simulink model "UAV_dinamica_pqr"  (R2014b)
settings: Solver=ode45  StartTime=0.0  StopTime=10.0  RelTol=1e-3
values from neighbouring files (symbols this model uses):
  Ir = 1e-3    (= 0.001)    [main_model1.m]    (also in main_model2.m; main_modelo_linear_v1.m = 0.01; main_modelo_linear_v2.m = 0.01; main_modelo_nao_linear_v1.m)
  Ixx = 1e-2    (= 0.01)    [main_model1.m]    (also in main_model2.m; main_modelo_linear_v1.m; main_modelo_linear_v2.m; main_modelo_nao_linear_v1.m)
  Iyy = 1e-2    (= 0.01)    [main_model1.m]    (also in main_model2.m; main_modelo_linear_v1.m; main_modelo_linear_v2.m; main_modelo_nao_linear_v1.m)
  Izz = 1.8e-2    (= 0.018)    [main_model1.m]    (also in main_model2.m; main_modelo_linear_v1.m; main_modelo_linear_v2.m; main_modelo_nao_linear_v1.m)
  Kd_rot = 0.01    [main_model1.m]    (also in main_model2.m; main_modelo_linear_v1.m = 0; main_modelo_linear_v2.m = 0; main_modelo_nao_linear_v1.m)
  Ki_rot = 1.0    (= 1)    [main_model1.m]    (also in main_model2.m; main_modelo_linear_v1.m = 0.5; main_modelo_linear_v2.m = 0.5; main_modelo_nao_linear_v1.m)
  Kp_rot = 10    [main_model1.m]    (also in main_model2.m; main_modelo_linear_v1.m = 1; main_modelo_linear_v2.m = 1; main_modelo_nao_linear_v1.m)
  p0 = 0    [main_model2.m]    (also in main_modelo_linear_v1.m; main_modelo_linear_v2.m; main_modelo_nao_linear_v2.m; modelo_naolinear.m)
  q0 = 0    [main_model2.m]    (also in main_modelo_linear_v1.m; main_modelo_linear_v2.m; main_modelo_nao_linear_v2.m; modelo_naolinear.m)
  r0 = 0    [main_model2.m]    (also in main_modelo_linear_v1.m; main_modelo_linear_v2.m; main_modelo_nao_linear_v2.m; modelo_naolinear.m)
libraries: simulink x3
settings Model: Creator=dferr  LastModifiedBy=dferr

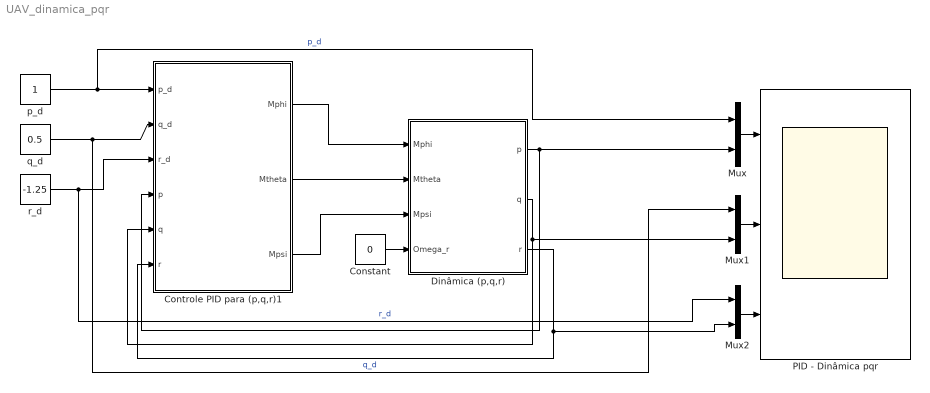
== system UAV_dinamica_pqr ==
  Constant : Constant  Value=0
  Controle PID para (p,q,r)1 : Subsystem
  Dinâmica (p,q,r) : Subsystem
      mask Display:
      | disp('(p,q,r)')
      | port_label('input',1,'Mphi')
      | port_label('input',2,'Mtheta')
      | port_label('input',3,'Mpsi')
      | port_label('input',4,'Omega_r')
      | port_label('output',1,'p')
      | port_label('output',2,'q')
      | port_label('output',3,'r')
  Mux : Mux  Inputs=2
  Mux1 : Mux  Inputs=2
  Mux2 : Mux  Inputs=2
  PID - Dinâmica pqr : Scope  NumInputPorts=3
      settings: YMin=-5~-5~-5  YMax=5~5~5
  p_d : Constant
  q_d : Constant  Value=0.5
  r_d : Constant  Value=-1.25
  wires:
  Controle PID para (p,q,r)1/1(Mphi) -> Dinâmica (p,q,r)/1(Mphi)
  Controle PID para (p,q,r)1/2(Mtheta) -> Dinâmica (p,q,r)/2(Mtheta)
  Controle PID para (p,q,r)1/3(Mpsi) -> Dinâmica (p,q,r)/3(Mpsi)
  Constant/1 -> Dinâmica (p,q,r)/4(Omega_r)
  r_d/1 -> Controle PID para (p,q,r)1/3(r_d), Mux2/1  "r_d"
  Mux1/1 -> PID - Dinâmica pqr/2
  Mux2/1 -> PID - Dinâmica pqr/3
  p_d/1 -> Mux/1, Controle PID para (p,q,r)1/1(p_d)  "p_d"
  Dinâmica (p,q,r)/1(p) -> Mux/2, Controle PID para (p,q,r)1/4(p)
  Mux/1 -> PID - Dinâmica pqr/1
  Dinâmica (p,q,r)/2(q) -> Mux1/2, Controle PID para (p,q,r)1/5(q)
  Dinâmica (p,q,r)/3(r) -> Mux2/2, Controle PID para (p,q,r)1/6(r)
  q_d/1 -> Mux1/1, Controle PID para (p,q,r)1/2(q_d)  "q_d"

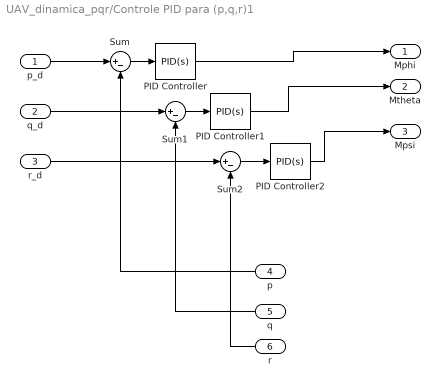
== system UAV_dinamica_pqr/Controle PID para (p,q,r)1 ==
  p_d : Inport
  q_d : Inport  Port=2
  r_d : Inport  Port=3
  p : Inport  Port=4
  q : Inport  Port=5
  r : Inport  Port=6
  PID Controller : simulink/Continuous/PID Controller  Controller=PID  TimeDomain=Continuous-time  SampleTime=-1  IntegratorMethod=Forward Euler  FilterMethod=Forward Euler  Form=Ideal  P=Kp_rot  I=Ki_rot  D=Kd_rot  N=100  InitialConditionSource=internal  InitialConditionForIntegrator=0  InitialConditionForFilter=0  ExternalReset=none  LimitOutput=off  UpperSaturationLimit=inf  LowerSaturationLimit=-inf  LinearizeAsGain=on  AntiWindupMode=none  Kb=1  TrackingMode=off  Kt=1  PParamMin=[]  PParamMax=[]  IParamMin=[]  IParamMax=[]  DParamMin=[]  DParamMax=[]  NParamMin=[]  NParamMax=[]  KbParamMin=[]  KbParamMax=[]  KtParamMin=[]  KtParamMax=[]  POutMin=[]  POutMax=[]  IOutMin=[]  IOutMax=[]  DOutMin=[]  DOutMax=[]  NOutMin=[]  NOutMax=[]  KbOutMin=[]  KbOutMax=[]  KtOutMin=[]  KtOutMax=[]  IntegratorOutMin=[]  IntegratorOutMax=[]  FilterOutMin=[]  FilterOutMax=[]  SumOutMin=[]  SumOutMax=[]  SumI1OutMin=[]  SumI1OutMax=[]  SumI2OutMin=[]  SumI2OutMax=[]  SumI3OutMin=[]  SumI3OutMax=[]  SumDOutMin=[]  SumDOutMax=[]  SaturationOutMin=[]  SaturationOutMax=[]  IntegratorContinuousStateAttributes=''  IntegratorStateMustResolveToSignalObject=off  IntegratorRTWStateStorageClass=Auto  FilterContinuousStateAttributes=''  FilterStateMustResolveToSignalObject=off  FilterRTWStateStorageClass=Auto  DifferentiatorICPrevScaledInput=0  DifferentiatorOutMin=[]  DifferentiatorOutMax=[]  UseFilter=on
  PID Controller1 : simulink/Continuous/PID Controller  Controller=PID  TimeDomain=Continuous-time  SampleTime=-1  IntegratorMethod=Forward Euler  FilterMethod=Forward Euler  Form=Ideal  P=Kp_rot  I=Ki_rot  D=Kd_rot  N=100  InitialConditionSource=internal  InitialConditionForIntegrator=0  InitialConditionForFilter=0  ExternalReset=none  LimitOutput=off  UpperSaturationLimit=inf  LowerSaturationLimit=-inf  LinearizeAsGain=on  AntiWindupMode=none  Kb=1  TrackingMode=off  Kt=1  PParamMin=[]  PParamMax=[]  IParamMin=[]  IParamMax=[]  DParamMin=[]  DParamMax=[]  NParamMin=[]  NParamMax=[]  KbParamMin=[]  KbParamMax=[]  KtParamMin=[]  KtParamMax=[]  POutMin=[]  POutMax=[]  IOutMin=[]  IOutMax=[]  DOutMin=[]  DOutMax=[]  NOutMin=[]  NOutMax=[]  KbOutMin=[]  KbOutMax=[]  KtOutMin=[]  KtOutMax=[]  IntegratorOutMin=[]  IntegratorOutMax=[]  FilterOutMin=[]  FilterOutMax=[]  SumOutMin=[]  SumOutMax=[]  SumI1OutMin=[]  SumI1OutMax=[]  SumI2OutMin=[]  SumI2OutMax=[]  SumI3OutMin=[]  SumI3OutMax=[]  SumDOutMin=[]  SumDOutMax=[]  SaturationOutMin=[]  SaturationOutMax=[]  IntegratorContinuousStateAttributes=''  IntegratorStateMustResolveToSignalObject=off  IntegratorRTWStateStorageClass=Auto  FilterContinuousStateAttributes=''  FilterStateMustResolveToSignalObject=off  FilterRTWStateStorageClass=Auto  DifferentiatorICPrevScaledInput=0  DifferentiatorOutMin=[]  DifferentiatorOutMax=[]  UseFilter=on
  PID Controller2 : simulink/Continuous/PID Controller  Controller=PID  TimeDomain=Continuous-time  SampleTime=-1  IntegratorMethod=Forward Euler  FilterMethod=Forward Euler  Form=Ideal  P=Kp_rot  I=Ki_rot  D=Kd_rot  N=100  InitialConditionSource=internal  InitialConditionForIntegrator=0  InitialConditionForFilter=0  ExternalReset=none  LimitOutput=off  UpperSaturationLimit=inf  LowerSaturationLimit=-inf  LinearizeAsGain=on  AntiWindupMode=none  Kb=1  TrackingMode=off  Kt=1  PParamMin=[]  PParamMax=[]  IParamMin=[]  IParamMax=[]  DParamMin=[]  DParamMax=[]  NParamMin=[]  NParamMax=[]  KbParamMin=[]  KbParamMax=[]  KtParamMin=[]  KtParamMax=[]  POutMin=[]  POutMax=[]  IOutMin=[]  IOutMax=[]  DOutMin=[]  DOutMax=[]  NOutMin=[]  NOutMax=[]  KbOutMin=[]  KbOutMax=[]  KtOutMin=[]  KtOutMax=[]  IntegratorOutMin=[]  IntegratorOutMax=[]  FilterOutMin=[]  FilterOutMax=[]  SumOutMin=[]  SumOutMax=[]  SumI1OutMin=[]  SumI1OutMax=[]  SumI2OutMin=[]  SumI2OutMax=[]  SumI3OutMin=[]  SumI3OutMax=[]  SumDOutMin=[]  SumDOutMax=[]  SaturationOutMin=[]  SaturationOutMax=[]  IntegratorContinuousStateAttributes=''  IntegratorStateMustResolveToSignalObject=off  IntegratorRTWStateStorageClass=Auto  FilterContinuousStateAttributes=''  FilterStateMustResolveToSignalObject=off  FilterRTWStateStorageClass=Auto  DifferentiatorICPrevScaledInput=0  DifferentiatorOutMin=[]  DifferentiatorOutMax=[]  UseFilter=on
  Sum : Sum  Inputs=|+-
  Sum1 : Sum  Inputs=|+-
  Sum2 : Sum  Inputs=|+-
  Mphi : Outport
  Mtheta : Outport  Port=2
  Mpsi : Outport  Port=3
  wires:
  p_d/1 -> Sum/1
  q_d/1 -> Sum1/1
  r/1 -> Sum2/2
  Sum2/1 -> PID Controller2/1
  PID Controller/1 -> Mphi/1
  r_d/1 -> Sum2/1
  q/1 -> Sum1/2
  p/1 -> Sum/2
  Sum1/1 -> PID Controller1/1
  PID Controller1/1 -> Mtheta/1
  Sum/1 -> PID Controller/1
  PID Controller2/1 -> Mpsi/1

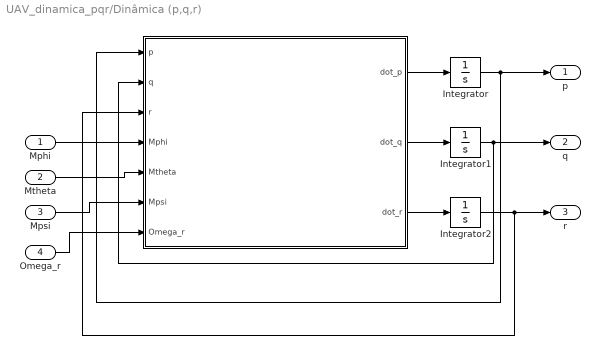
== system UAV_dinamica_pqr/Dinâmica (p,q,r) ==
  Mphi : Inport
  Mtheta : Inport  Port=2
  Mpsi : Inport  Port=3
  Omega_r : Inport  Port=4
  "  " : Subsystem
      mask Display:
      | disp('Dinâmica Rotacional no Corpo')
      | port_label('input',1,'p')
      | port_label('input',2,'q')
      | port_label('input',3,'r')
      | port_label('input',4,'Mphi')
      | port_label('input',5,'Mtheta')
      | port_label('input',6,'Mpsi')
      | port_label('input',7,'Omega_r')
      | port_label('output',1,'dot_p')
      | port_label('output',2,'dot_q')
      | port_label('output',3,'dot_r')
  Integrator : Integrator  InitialCondition=p0
  Integrator1 : Integrator  InitialCondition=q0
  Integrator2 : Integrator  InitialCondition=r0
  p : Outport
  q : Outport  Port=2
  r : Outport  Port=3
  wires:
  "  "/3(dot_r) -> Integrator2/1
  Integrator2/1 -> r/1, "  "/3(r)
  "  "/2(dot_q) -> Integrator1/1
  "  "/1(dot_p) -> Integrator/1
  Integrator1/1 -> q/1, "  "/2(q)
  Integrator/1 -> p/1, "  "/1(p)
  Mpsi/1 -> "  "/6(Mpsi)
  Mtheta/1 -> "  "/5(Mtheta)
  Mphi/1 -> "  "/4(Mphi)
  Omega_r/1 -> "  "/7(Omega_r)

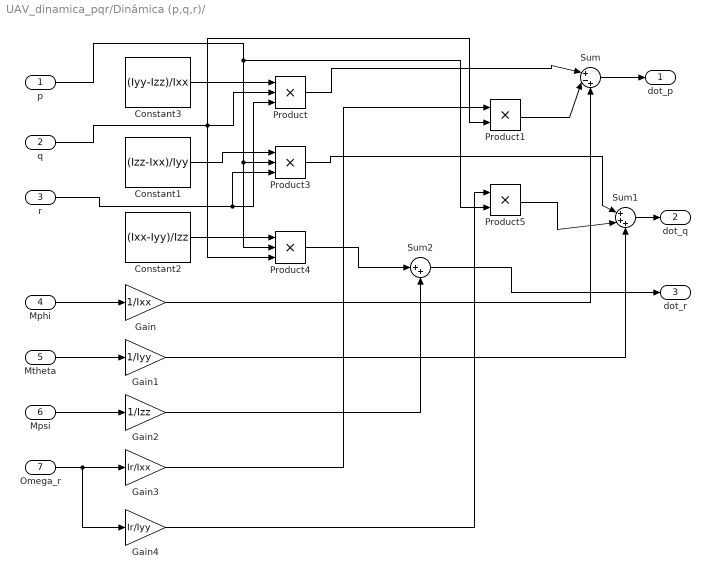
== system UAV_dinamica_pqr/Dinâmica (p,q,r)/   ==
  p : Inport
  q : Inport  Port=2
  r : Inport  Port=3
  Mphi : Inport  Port=4
  Mtheta : Inport  Port=5
  Mpsi : Inport  Port=6
  Omega_r : Inport  Port=7
  Constant1 : Constant  Value=(Izz-Ixx)/Iyy
  Constant2 : Constant  Value=(Ixx-Iyy)/Izz
  Constant3 : Constant  Value=(Iyy-Izz)/Ixx
  Gain : Gain  Gain=1/Ixx
  Gain1 : Gain  Gain=1/Iyy
  Gain2 : Gain  Gain=1/Izz
  Gain3 : Gain  Gain=Ir/Ixx
  Gain4 : Gain  Gain=Ir/Iyy
  Product : Product  Inputs=3
  Product1 : Product
  Product3 : Product  Inputs=3
  Product4 : Product  Inputs=3
  Product5 : Product
  Sum : Sum  Inputs=|+-+
  Sum1 : Sum  Inputs=|+++
  Sum2 : Sum  Inputs=|++
  dot_p : Outport
  dot_q : Outport  Port=2
  dot_r : Outport  Port=3
  wires:
  Product/1 -> Sum/1
  Sum/1 -> dot_p/1
  Constant1/1 -> Product3/1
  Constant3/1 -> Product/1
  r/1 -> Product3/3, Product/3
  Gain1/1 -> Sum1/3
  Mtheta/1 -> Gain1/1
  p/1 -> Product5/2, Product4/2, Product3/2
  Gain/1 -> Sum/3
  q/1 -> Product4/3, Product1/2, Product/2
  Product4/1 -> Sum2/1
  Mpsi/1 -> Gain2/1
  Constant2/1 -> Product4/1
  Sum2/1 -> dot_r/1
  Gain4/1 -> Product5/1
  Product1/1 -> Sum/2
  Product3/1 -> Sum1/1
  Gain2/1 -> Sum2/2
  Gain3/1 -> Product1/1
  Product5/1 -> Sum1/2
  Mphi/1 -> Gain/1
  Sum1/1 -> dot_q/1
  Omega_r/1 -> Gain4/1, Gain3/1
